simulink model "VC_v1p1"  (R2022b)
settings: Solver=VariableStepAuto  StartTime=0.0  StopTime=inf  FixedStep=1/100  MaxStep=ts  RelTol=1e-3
InitFcn:
  | init_car
  | init_par
values from neighbouring files (symbols this model uses):
  east0 = EWP(1)    [run_VC_bench.m]
  g = 9.81    [init_car.m]
  north0 = NWP(1)    [run_VC_bench.m]
  NUM_WP = length(NWP)    [run_VC_bench.m]
  psi0 = (pi/180)*HWP(1)    [run_VC_bench.m]
  ts = 1/fs    (= 0.01)    [init_car.m]
  vcg0 = 0    [run_VC_bench.m]
  WPT_MTX = [NWP,EWP,HWP,VWP,KWP,SWP]    [run_VC_bench.m]
undefined symbols (not defined in the file or in its folder): car, EWP, NWP, par, ZWP
libraries: simulink x9, matrix_library x6
(part 3 of 3)

== matlab function VC_v1p1/Vehicle_Controller/Lateral Control/Lateral Controller/Calculate control limits/Calculate Curvature Rate and Steering Limits based on vehicle speed using manufacturer data ==
  data: thetadotmax output; thetamax output; delta_s output; kmax output; kpmax output; vcar input; vdead input; ts input; kappa2theta input
function [thetadotmax, thetamax, delta_s, kmax, kpmax] = ...
    speed_based_limits(vcar, vdead, ts, kappa2theta)
%
%  theta = steering wheel angle (deg)
%  delta = front wheel angle (rad)
%  kappa = curvature of path (rad/m)
%
%  thetadotmax = maximumm allowable steering wheel rate (deg/s)
%  thetamax = maximum allowable steering wheel angle (deg)
%  delta_s = distance along path that car moves in one time step (m)
%  kmax = maximum curvature based on published limits (rad/m)
%  kpmax = maximum curvature rate based on published limits (rad/m/m)
%
%  vcar = car velocity (m/s)
%  vdead = deadzone velocity (m/s)
%  ts = sample period (sec)
%  kappa2theta = assumed linear scale factor between kappa and theta

%  This function computes the maximum curvature rate and the max theta at a
%  given vehicle speed based on GM published limits.
%
%  k' = dk/ds [rad/m^2]      vcar = ds/dt [m/s]
%
%  delta[deg] = theta2delta * theta[deg]
%
%  theta[deg] = k2theta * k[rad/m]
%
%  delta[rad] = k2delta * k[rad/m]
%
%  dk    d( theta )      1      (dtheta/dt)        1        (dtheta)
%  -- = ----------- = ------- * ----------- = ----------- * --------
%  ds   ds(k2theta)   k2theta   (  ds/dt  )   k2theta * v   (  dt  )
%
%  Check units:
%     dtheta/dt[deg/sec]
%     k2theta[deg-m/rad] * v[m/s] -> [deg-m^2/rad-s]
%
%  Last Updated:  1/26/2023

%  --initialize local persistent variables

persistent KPH THETAMAX THETADOTMAX NLUT mps2kph

if isempty(KPH)
    %  --define the GM limits on steering rate (lookup tables)
    KPH = [0 15 20 30 35 45 50 65 200];     % kilometers/hour
    THETAMAX = [531 531 475 375 325 235 100 75 10];     % degrees
    THETADOTMAX = [600 600 600 600 400 200 140 95 50];  % degrees/sec
    NLUT = 9;  % number of elements in the LUTs
    
    %  --define the conversion constants
    mps2kph = 3.6;          % kph(ki/hour) = mps2kph * mps(m/s)    
end


%  --evaluate the limits for the input speed

kph = mps2kph * abs(vcar);


%  --interpolate the LUT for the given input speed

if (kph <= KPH(1))
    %  --saturate at the minimum speed in the LUT
    thetadotmax = THETADOTMAX(1);   % (deg/s)
    thetamax = THETAMAX(1);         % (deg)
    
elseif (kph >= KPH(NLUT))
    %  --saturate at the maximum speed in the LUT
    thetadotmax = THETADOTMAX(NLUT);   % (deg/s)
    thetamax = THETAMAX(NLUT);         % (deg)
    
else
    %  --find the interval containing this speed
    index = 2;
    while (kph > KPH(index))
        index = index + 1;  % always points to the upper end of the interval
    end
    
    %  --interpolate the values
    ratio = (kph - KPH(index-1)) / (KPH(index) - KPH(index-1));
    
    thetadotmax = THETADOTMAX(index-1) + ...
        ratio * (THETADOTMAX(index) - THETADOTMAX(index-1));  % (deg/s)
    
    thetamax = THETAMAX(index-1) + ...
        ratio * (THETAMAX(index) - THETAMAX(index-1));  % (deg)
end


%  --compute the maximum curvature based on speed

kmax = thetamax / kappa2theta;


%  --convert thetadotmax (deg/s) to kpmax (rad/m^2)

if (abs(vcar) > 0.1)
    kpmax = thetadotmax / (kappa2theta * vcar);   % (rad/m^2)
else
    %  --saturate to avoid the zero-divide
    kpmax = THETADOTMAX(1) / (kappa2theta * 0.1);   % (rad/m^2);
end


%  --determine how far vehicle traveled in one time step

if (abs(vcar) < vdead)
    %  --car is effectively stopped
    delta_s = 0;
else
    %  --car is moving
    delta_s = abs(vcar) * ts;
end

return

== matlab function VC_v1p1/Vehicle_Controller/Lateral Control/Lateral Controller/Calculate control limits/Calculate Curvature Rate Limits based on geometry ==
  data: kcar input; R input; kpmax_geo output; kpmin_geo output
function [kpmax_geo,kpmin_geo] = geometry_based_limits(kcar, R)
%
%  This is a gateway function to get_kp_limit.m

[kpmax_geo,kpmin_geo] = get_kp_limit(kcar,R);

return

== matlab function VC_v1p1/Vehicle_Controller/Lateral Control/Lateral Controller/Calculate the next desired Curvature Rate ==
  data: kcar input size=1; kpmax input size=1; kpmin input size=1; R input size=1; psi input size=1; Ncar input size=1; Ntarget input size=1; Ecar input size=1; Etarget input size=1; kpdes output size=1
function kpdes = optimal_curvature_rate(kcar, kpmax, kpmin, R, ...
    psi, Ncar, Ntarget, Ecar, Etarget)

%  This is a gateway function to get_opt_curvature_rate.m

maxiter = 10;
tol = 1e-3;

kpdes  = get_opt_curvature_rate(kcar, kpmax, kpmin, R, ...
    psi, Ncar, Ntarget, Ecar, Etarget, maxiter, tol);

return

== matlab function VC_v1p1/Vehicle_Controller/Longitudinal Control/Longitudinal Controller/velocity feedback pre-processor/MATLAB Function ==
  data: speed_mode input; vref input; vcar input; vdes output; alat input; along input; ts input; max_speed input; max_alat input; fbreak_vref input; verror output; vdead input; car_is_stopped output
function [vdes,verror,car_is_stopped]  = prefilter_vref(speed_mode, ...
    vref,vcar,alat,along, ...
    ts,max_speed,max_alat,fbreak_vref,vdead)

%  vdes = final desired reference velocity for control (m/s)
%  verror = velocity error for control (m/s)
%  car_is_stopped = boolean indicating that the car is not moving
%
%  speed_mode = operating mode for speed control
%    * = both torque and brake commands are set to zero
%    1 = brake hold mode (max brake and no torque)
%    2 = use internal torque and brake signals
%    3 = use external torque and brake signals
%  vcar = current car velocity (m/s)
%  vref = current input reference velocity (m/s)
%  alat = current lateral acceleration (m/s/s)
%  along = current longitudinal acceleration (m/s/s) [not yet used]
%  ts = sample period (sec)
%  max_speed = maximum vehicle speed (m/s)
%  max_alat = maximum lateral acceleration (m/s/s)
%  fbreak_vref = break frequency (Hz) of 1st order low-pass filter
%  vdead = deadzone velocity (m/s)

%  --define persistent local variables
persistent VDES VERROR LAST_SPEED_MODE LPFA LPFB CAR_IS_STOPPED
persistent VREF LAST_VREF_IN LAST_VREF_OUT
persistent LAST_ALAT_IN LAST_ALAT_OUT
persistent soft_start_state deltaVREF startup_accel soft_start_count
if (isempty(VDES))
    VDES = 0;
    VERROR = 0;
    CAR_IS_STOPPED = 1;
    LAST_SPEED_MODE = 0;
    VREF = 0;
    LAST_VREF_IN = 0;
    LAST_VREF_OUT = 0;
    LAST_ALAT_IN = 0;
    LAST_ALAT_OUT = 0;
    soft_start_state = 0;
    startup_accel = 0.5;  % m/s/s
    deltaVREF = startup_accel * ts;
    soft_start_count = 0;

    %  --compute low-pass vref filter coefficients
    w = 2*pi*fbreak_vref;   % break frequency for vref (rad/s)
    LPFA = (w*ts-2)/(w*ts+2);  % numerator coefficient
    LPFB = (w*ts)/(w*ts+2);    % denominator coefficient
end

%  --check for a mode transition
if (speed_mode ~= LAST_SPEED_MODE)
    %  --recompute low-pass vref filter coefficients
    w = 2*pi*fbreak_vref;   % break frequency for vref (rad/s)
    LPFA = (w*ts-2)/(w*ts+2);  % numerator coefficient
    LPFB = (w*ts)/(w*ts+2);    % denominator coefficient

    %  --reset local signals
    VDES = 0;
    VERROR = 0;
    CAR_IS_STOPPED = 1;
    VREF = 0;
    LAST_VREF_IN = 0;
    LAST_VREF_OUT = 0;
    LAST_ALAT_IN = 0;
    LAST_ALAT_OUT = 0;
    soft_start_state = 0;
    deltaVREF = startup_accel * ts;
    soft_start_count = 0;
end


%  --check to see if car is moving
if (abs(vcar) < vdead)
    %  --car is not moving
    CAR_IS_STOPPED = 1;
else
    %  --car is still moving
    CAR_IS_STOPPED = 0;
end


%  --only process for mode 2 (autonomous speed control)
if (speed_mode == 2)
    %  --filter the absolute lateral acceleration input
    alat_out = LPFB * (abs(alat) + LAST_ALAT_IN) - LPFA * LAST_ALAT_OUT;
    LAST_ALAT_OUT = alat_out;
    LAST_ALAT_IN = abs(alat);


    %  --adjust the upper speed limit based on lateral acceleration
    if (CAR_IS_STOPPED == 1)
        %  --car is not moving so just use max speed
        vmax = max_speed;
        soft_start_count = 0;  % reset soft_start counter

    else
        %  --car is moving so check lateral acceleration limit
        if (abs(alat_out) > max_alat)
            %  --lat acceleration exceeded limits (too high)
            %    calculate vmax based on max alat
            %    (vmax/vcar)^2 = (max_alat/alat)
            vmax = abs(vcar) * sqrt(max_alat / abs(alat_out));

            if (vmax > max_speed)
                %  --saturate the velocity limit at the max speed limit
                vmax = max_speed;
            end
        else
            %  --lat acceleration is within limits
            vmax = max_speed;
        end
    end


    %  --soft start state machine
    switch soft_start_state
        case 0  %  --waiting for start
            if (vref > 0)
                %  --enter soft-start mode
                VREF = 0;
                soft_start_state = 2;
            end

            LAST_VREF_IN = VREF;
            LAST_VREF_OUT = VREF;
            soft_start_count = 0;

        case 1  %  --ramp up the ref velocity at a fixed rate for 1 sec
            if (soft_start_count < 200)
                %  --counter has not yet expired
                VREF = VREF + deltaVREF;
                soft_start_count = soft_start_count + 1;
            else
                %  --counter has expired
                soft_start_state = 2;
            end

        case 2  %  --ramp up the reference velocity at a fixed rate
            if (VREF < min(vref,vmax))
                %  --reference velocity is still below the command
                VREF = VREF + deltaVREF;
            else
                %  --reference velocity has reached the command
                soft_start_state = 3;
            end

        case 3  %  --track the actual reference input velocity now
            if (CAR_IS_STOPPED == 1)
                %  --return to wait state
                soft_start_state = 0;
            else
                %  --normal operation
                VREF = min(vref,vmax);
            end

        otherwise
            %  --should not be here
            soft_start_state = 0;
    end


    %  --low-pass filter the reference velocity
    VDES = LPFB * (VREF + LAST_VREF_IN) - LPFA * LAST_VREF_OUT;
    LAST_VREF_OUT = VDES;  % desired reference velocity
    LAST_VREF_IN = VREF;


    %  --compute the velocity feedback error for control
    VERROR = VDES - vcar;

else
    %  --not doing speed control so zero the outputs
    VDES = 0;
    VERROR = 0;
    soft_start_state = 0;
end


%  --transfer outputs
vdes = VDES;
verror = VERROR;
car_is_stopped = CAR_IS_STOPPED;
LAST_SPEED_MODE = speed_mode;

return

== matlab function VC_v1p1/Vehicle_Controller/Lateral Control/Lateral Controller/Calculate Steering Command/Integrate Curvature Rate and compute next Steering Command ==
  data: steer_cmd output; steer_mode input; thetadotmax input; thetamax input; delta_s input; kmax input; kpdes input; kappa2theta input; ts input; max_steer input; min_steer input; max_delta_steer input; kdes output
function [steer_cmd,kdes] = integrate_curv_rate(steer_mode, ...
    thetadotmax, thetamax, delta_s, kmax, kpdes, ...
    kappa2theta, ts, max_steer, min_steer, max_delta_steer)

%  steer_cmd = output steering wheel command position (deg)
%
%  steer_mode = operating mode selector for steering
%    * = steer command set to zero
%    1 = hold steer signal at last value
%    2 = use internal steer signal
%    3 = use external steer signal
%  thetadotmax = maximum steering wheel rate (deg/s)
%  thetamax = maximum steering wheel position (deg)
%  delta_s = distance car travels over one time step (m)
%  kmax = maximum curvature (rad/m)
%  kpdes = desired curvature rate (rad/m/m)
%  kappa2theta = conversion factor between curvature and steering wheel angle
%  ts = sample period (sec)
%  max_steer = maximum allowable steering wheel angle (deg)
%  min_steer = minimum allowable steering wheel angle (deg)
%  max_delta_steer = maximum change in steering wheel command angle (deg)

%  --define local persistent variables
persistent KDES STEER_CMD LAST_STEER_MODE LAST_STEER_CMD
if (isempty(KDES))
    %  --initialize local persistent variables at compile time
    KDES = 0;
    STEER_CMD = 0;
    LAST_STEER_MODE = 0;
    LAST_STEER_CMD = 0;
end


%  --check for steer mode

switch steer_mode
    case 1
        %  --halt the integration, hold output value constant
        % do nothing here

    case 2
        %  --reset integrator on mode transition
        if (steer_mode ~= LAST_STEER_MODE)
            KDES = 0;
        end

        %  --integrate the curvature rate to get the desired curvature
        KDES = KDES + kpdes * delta_s;  % (rad/m)


        %  --saturate the desired curvature
        if (KDES > kmax)
            %  --saturate at upper limit
            KDES = kmax;
        elseif (KDES < -kmax)
            %  --saturate at lower limit
            KDES = -kmax;
        end

    otherwise
        KDES = 0;
end


%  --compute the next steering command
STEER_CMD = KDES * kappa2theta;  % (deg)


%  --compute the max delta steer
MAX_delta_steer = thetadotmax * ts;  % (deg) = (deg/s) * (s)
MAX_delta_steer = min(MAX_delta_steer, max_delta_steer);


%  --rate limit the steering command
if (STEER_CMD > (LAST_STEER_CMD + MAX_delta_steer))
    %  --delta steer is too large in the positive direction
    STEER_CMD = LAST_STEER_CMD + MAX_delta_steer;

elseif (STEER_CMD < (LAST_STEER_CMD - MAX_delta_steer))
    %  --delta steer is too large in the negative direction
    STEER_CMD = LAST_STEER_CMD - MAX_delta_steer;
end


%  --choose conservztive steering command limits
if (thetamax < max_steer)
    MAX_steer = thetamax;
else
    MAX_steer = max_steer;
end
if (min_steer < -thetamax)
    MIN_steer = -thetamax;
else
    MIN_steer = min_steer;
end

%  --saturate the steering command
if (STEER_CMD > MAX_steer)
    STEER_CMD = MAX_steer;
elseif (STEER_CMD < MIN_steer)
    STEER_CMD = MIN_steer;
end


%  --transfer local variables
steer_cmd = STEER_CMD;
kdes = KDES;
LAST_STEER_CMD = steer_cmd;
LAST_STEER_MODE = steer_mode;

return

== matlab function VC_v1p1/Vehicle_Controller/Longitudinal Control/Longitudinal Controller/Speed Controller/PID Controller for tracking speed ==
  data: speed_mode input; torque_cmd output; pitch input; verror input; ts input; max_drv_torque input; max_delta_torque input; min_brk_torque input; max_delta_brake input; kp input; ki input; kd input; kff input; fbreak_diff input; fbreak_fflpf input
function torque_cmd  = speed_controller( ...
    speed_mode,pitch,verror,ts, ...
    max_drv_torque,max_delta_torque, ...
    min_brk_torque,max_delta_brake, ...
    kp,ki,kd,kff,fbreak_diff,fbreak_fflpf)

%  torque_cmd = final output torque command (Nm)
%
%  speed_mode = operating mode for speed control
%    * = both torque and brake commands are set to zero
%    1 = brake hold mode (max brake and no torque)
%    2 = use internal torque and brake signals
%  pitch = pitch angle of the vehicle (rad)
%  verror = velocity error for speed control (m/s)
%  ts = sample period (sec)
%  max_drv_torque = maximum allowable drive torque (Nm)
%  min_drv_torque = minimum allowable drive torque (Nm)
%  max_delta_torque = maximum allowable change in drive torque (Nm)
%  max_brk_torque = maximum allowable brake torque (Nm)
%  min_brk_torque = minimum allowable brake torque (Nm)
%  max_delta_brake = maximum allowable change in brake torque (Nm)
%  kp = proportional feedback gain
%  ki = integral feedback gain
%  kd = derivative feedback gain
%  kff = feedforward gain for pitch angle compensation
%  fbreak_diff = 1st order break frequency (Hz) for differentiator
%  fbreak_fflpf = 1st order break frequency (Hz) for feedforward LPF

%  --define the local persistent variables
persistent LPFA LPFB DIFFA DIFFB PROP_ERROR INTE_ERROR DERIV_ERROR
persistent LAST_SPEED_MODE LAST_TORQUE_CMD
persistent LAST_VERROR LAST_PITCH PITCH_OUT
if (isempty(LAST_SPEED_MODE))
    %  --initialize local persistent variables
    LAST_SPEED_MODE = 0;
    PROP_ERROR = 0;
    INTE_ERROR = 0;
    DERIV_ERROR = 0;
    LAST_VERROR = 0;
    LAST_PITCH = 0;
    PITCH_OUT = 0;
    LAST_TORQUE_CMD = 0;

    %  --compute low-pass (pitch) filter coefficients
    w = 2*pi*fbreak_fflpf;       % break frequency for vref (rad/s)
    LPFA = (w*ts-2)/(w*ts+2);  % numerator coefficient
    LPFB = (w*ts)/(w*ts+2);    % denominator coefficient

    %  --compute the high-pass (differentiator) filter coefficients
    w = 2*pi*fbreak_diff;       % break frequency (rad/s)
    DIFFA = (w*ts-2)/(w*ts+2);  % discrete-time denominator coefficient
    DIFFB = (2*w)/(w*ts+2);     % discrete-time numerator coefficient
end


%  --check for a mode transition
if (speed_mode ~= LAST_SPEED_MODE)
    %  --recompute low-pass (pitch) filter coefficients
    w = 2*pi*fbreak_fflpf;       % break frequency for vref (rad/s)
    LPFA = (w*ts-2)/(w*ts+2);  % numerator coefficient
    LPFB = (w*ts)/(w*ts+2);    % denominator coefficient

    %  --recompute the high-pass (differentiator) filter coefficients
    w = 2*pi*fbreak_diff;       % break frequency (rad/s)
    DIFFA = (w*ts-2)/(w*ts+2);  % discrete-time denominator coefficient
    DIFFB = (2*w)/(w*ts+2);     % discrete-time numerator coefficient

    %  --reset local persistent variables
    PROP_ERROR = 0;
    INTE_ERROR = 0;
    DERIV_ERROR = 0;
    LAST_VERROR = 0;
    LAST_PITCH = 0;
    PITCH_OUT = 0;
    LAST_TORQUE_CMD = 0;
end


%  --only process for mode 2 (autonomous speed control)
if (speed_mode == 2)
    %  --evaluate the proportional control term
    PROP_ERROR = kp * verror;


    %  --evaluate and saturate the integral control term
    INTE_ERROR = INTE_ERROR + ki * verror;
    if (INTE_ERROR > max_drv_torque)
        %  --extreme upper limit
        INTE_ERROR = max_drv_torque;
    elseif (INTE_ERROR < min_brk_torque)
        %  --extreme lower limit
        INTE_ERROR = min_brk_torque;
    end


    %  --evaluate the derivative control term
    DERIV_ERROR = (kd * DIFFB * (verror - LAST_VERROR)) - DIFFA * DERIV_ERROR;
    LAST_VERROR = verror;


    %  --low-pass filter the pitch angle
    PITCH_OUT = LPFB * (pitch - LAST_PITCH) - LPFA * PITCH_OUT;
    LAST_PITCH = pitch;

    
    %  --compute the total PID control signal with FF pitch compensation
    TORQUE_CMD = PROP_ERROR + INTE_ERROR + DERIV_ERROR + kff * sin(PITCH_OUT);


    %  --rate limit the TORQUE_CMD value
    if (TORQUE_CMD > 0)
        %  --use throttle torque limits
        if (TORQUE_CMD > (LAST_TORQUE_CMD + max_delta_torque))
            %  --delta torque is too large in the positive direction
            TORQUE_CMD = LAST_TORQUE_CMD + max_delta_torque;

%         elseif (TORQUE_CMD < (LAST_TORQUE_CMD - max_delta_torque))
%             %  --delta torque is too large in the negative direction
%             TORQUE_CMD = LAST_TORQUE_CMD - max_delta_torque;
        end

        %  --saturate the final torque command
        if (TORQUE_CMD > max_drv_torque)
            %  --requested torque exceeds upper limit
            TORQUE_CMD = max_drv_torque;
        end

    else
        %  --use brake torque limits
        if (TORQUE_CMD > (LAST_TORQUE_CMD + max_delta_brake))
            %  --delta torque is too large in the positive direction
            TORQUE_CMD = LAST_TORQUE_CMD + max_delta_brake;

%         elseif (TORQUE_CMD < (LAST_TORQUE_CMD - max_delta_brake))
%             %  --delta torque is too large in the negative direction
%             TORQUE_CMD = LAST_TORQUE_CMD - max_delta_brake;
        end
        
        %  --saturate the final torque command
        if (TORQUE_CMD < min_brk_torque)
            %  --requested torque exceeds upper limit
            TORQUE_CMD = min_brk_torque;
        end

    end

else
    %  --all other speed_mode values have zero torque output
    TORQUE_CMD = 0;
end


%  --save the previous local TORQUE_CMD and BRAKE_CMD values
LAST_TORQUE_CMD = TORQUE_CMD;
LAST_SPEED_MODE = speed_mode;


%  --transfer local signals to the outputs
torque_cmd = TORQUE_CMD;

return

== matlab function VC_v1p1/Vehicle_Controller/Longitudinal Control/Longitudinal Controller/Speed Controller/Compensate brake path ==
  data: speed_mode input; torque_cmd input; throttle_cmd output; ts input; wT input; zT input; wB input; zB input; brake_cmd output; min_brk_torque input
function [throttle_cmd,brake_cmd] = lead_compensator(speed_mode, ...
    torque_cmd, ts, wT, zT, wB, zB, min_brk_torque)

%  throttle_cmd = final torque (throttle) command signal (Nm)
%  brake_cmd = lead-compensated brake command signal (Nm)
%
%  speed_mode = operating mode for speed control
%  torque_cmd = net input throttle command (Nm)
%  ts = sample period (sec)
%  wT = 2nd order natural frequency (rad/s) of torque dynamics
%  zT = damping ratio of torque dynamics
%  wB = 2nd order natural frequency (rad/s) of brake dynamics
%  zB = damping ratio of brake dynamics


%  --define  local persistent variables
persistent LAST_SPEED_MODE B0 B1 B2 A1 A2 ykm1 ykm2 ukm1 ukm2
persistent THROTTLE_CMD BRAKE_CMD
if (isempty(LAST_SPEED_MODE))
    %  --initialize local persistent variables
    LAST_SPEED_MODE = 0;
    ykm1 = 0;
    ykm2 = 0;
    ukm1 = 0;
    ukm2 = 0;
    THROTTLE_CMD = 0;
    BRAKE_CMD = 0;

    %  --initialize lead filter coefficients
    A0 = wB^2*(4*ts*wT*zT + ts^2*wT^2 + 4);
    A1 = wB^2*(2*ts^2*wT^2 - 8) / A0;
    A2 = wB^2*(ts^2*wT^2 - 4*ts*wT*zT + 4) / A0;
    B0 = wT^2*(4*ts*wB*zB + ts^2*wB^2 + 4) / A0;
    B1 = wT^2*(2*ts^2*wB^2 - 8) / A0;
    B2 = wT^2*(ts^2*wB^2 - 4*ts*wB*zB + 4) / A0;
end


%  --check for a mode change
if (speed_mode ~= LAST_SPEED_MODE)
    %  --reinitialize local persistent variables
    ykm1 = 0;
    ykm2 = 0;
    ukm1 = 0;
    ukm2 = 0;
    THROTTLE_CMD = 0;
    BRAKE_CMD = 0;

    %  --initialize lead filter coefficients
    A0 = wB^2*(4*ts*wT*zT + ts^2*wT^2 + 4);
    A1 = wB^2*(2*ts^2*wT^2 - 8) / A0;
    A2 = wB^2*(ts^2*wT^2 - 4*ts*wT*zT + 4) / A0;
    B0 = wT^2*(4*ts*wB*zB + ts^2*wB^2 + 4) / A0;
    B1 = wT^2*(2*ts^2*wB^2 - 8) / A0;
    B2 = wT^2*(ts^2*wB^2 - 4*ts*wB*zB + 4) / A0;
end


%  --only process torque/brake split when mode=2 (autonomous speed)

if (speed_mode == 1)
    %  --apply max brake torque in RDY_BRAKE mode
    BRAKE_CMD = min_brk_torque;
    THROTTLE_CMD = 0;

elseif (speed_mode == 2)
    %  --determine if torque input is for throttle or brake
    if (torque_cmd > 0)
        %  --process input torque_cmd as a throttle command
        THROTTLE_CMD = torque_cmd;
        BRAKE_CMD = 0;
        ykm1 = 0;
        ykm2 = 0;
        ukm1 = 0;
        ukm2 = 0;

    else
        %  --process input torque_cmd as a brake command
        THROTTLE_CMD = 0;

        %  --evaluate the lead filter with the next brake_cmd input
        BRAKE_CMD = - A1*ykm1 - A2*ykm2 + B0*torque_cmd + B1*ukm1 + B2*ukm2;

        %  --saturate the lead filter output (brake_cmd can never be positive)
        if (BRAKE_CMD > 0), BRAKE_CMD = 0; end

        %  --shift data for the next time step
        ykm2 = ykm1;
        ykm1 = BRAKE_CMD;   % previous output
        ukm2 = ukm1;
        ukm1 = torque_cmd;  % previous input
    end

else
    %  --zero all internal states and outputs
    ykm1 = 0;
    ykm2 = 0;
    ukm1 = 0;
    ukm2 = 0;
    THROTTLE_CMD = 0;
    BRAKE_CMD = 0;
end


%  --transfer outputs
LAST_SPEED_MODE = speed_mode;
throttle_cmd = THROTTLE_CMD;
brake_cmd = BRAKE_CMD;

return;

== matlab function VC_v1p1/Vehicle_Controller/Lateral Control/Lateral Controller/Calculate Steering Command/MATLAB Function ==
  data: steer_mode input; steer_cmd input; ts input; steer_lead output; fz_lead input; zz_lead input; fp_lead input
function steer_lead = lead_compensator(steer_mode,steer_cmd,ts,...
    fz_lead,zz_lead,fp_lead)
%  This function implements a 3rd order IIR filter using a Direct-Form II
%  structure.  This is a lead filter designed specifically to
%  compensate the steering command signal.
%
%  The Laplace-domain transfer function is:
%
%  y(s)     wp^3     (s^2 + 2*zz*wz*s + wz^2)   -> two complex zeros
%  ---- = -------- * ------------------------
%  x(s)   (s+wp)^3            wz^2              -> three real poles
%
%  The equivalent Z-domain transfer function is:
%
%  y(z)   b0*z^3 + b1*z^2 + b2*z + b3
%  ---- = ---------------------------
%  x(z)     z^3 + a1*z^2 + a2*z + a3
%
%  steer_cmd = input sample to the filter at time step k
%  ts = sample period (sec)
%  fz_lead = 2nd order zero frequency (Hz)
%  zz_lead = 2nd order zero damping ratio (nondim)
%  fp_lead = 1st order pole frequency (Hz)
%  steer_mode = operational mode for steer control
%  steer_lead = output sample from the filter at time step k
%  
%  Last Updated:  1/26/2023

%  --define local persistent variables
persistent LAST_STEER_MODE A1 A2 A3 B0 B1 B2 B3 LAST_STEER_LEAD
persistent ykm1 ykm2 ykm3 ukm1 ukm2 ukm3
if (isempty(LAST_STEER_MODE))
    %  --initialize local persistent variables
    LAST_STEER_MODE = 0;
    LAST_STEER_LEAD = 0;
    ykm1 = 0; ykm2 = 0; ykm3 = 0;
    ukm1 = 0; ukm2 = 0; ukm3 = 0;

    %  --initialize lead filter coefficients
    wz = 2*pi*fz_lead;
    zz = zz_lead;
    wp = 2*pi*fp_lead;

    A0 = (wz^2*(ts*wp + 2)^3);
    A1 = (3*wz^2*(ts*wp - 2)*(ts*wp + 2)^2) / A0;
    A2 = (3*wz^2*(ts*wp - 2)^2*(ts*wp + 2)) / A0;
    A3 = (wz^2*(ts*wp - 2)^3) / A0;
    B0 = (ts*wp^3*(4*ts*wz*zz + ts^2*wz^2 + 4)) / A0;
    B1 = (ts*wp^3*(3*ts^2*wz^2 + 4*ts*wz*zz - 4)) / A0;
    B2 = (-ts*wp^3*(4*ts*wz*zz - 3*ts^2*wz^2 + 4)) / A0;
    B3 = (ts*wp^3*(ts^2*wz^2 - 4*ts*wz*zz + 4)) / A0;
end


%  --check for a mode change
if (steer_mode ~= LAST_STEER_MODE)
    %  --reinitialize local persistent variables
    LAST_STEER_LEAD = 0;
    ykm1 = 0; ykm2 = 0; ykm3 = 0;
    ukm1 = 0; ukm2 = 0; ukm3 = 0;

    %  --initialize lead filter coefficients
    wz = 2*pi*fz_lead;
    zz = zz_lead;
    wp = 2*pi*fp_lead;

    A0 = (wz^2*(ts*wp + 2)^3);
    A1 = (3*wz^2*(ts*wp - 2)*(ts*wp + 2)^2) / A0;
    A2 = (3*wz^2*(ts*wp - 2)^2*(ts*wp + 2)) / A0;
    A3 = (wz^2*(ts*wp - 2)^3) / A0;
    B0 = (ts*wp^3*(4*ts*wz*zz + ts^2*wz^2 + 4)) / A0;
    B1 = (ts*wp^3*(3*ts^2*wz^2 + 4*ts*wz*zz - 4)) / A0;
    B2 = (-ts*wp^3*(4*ts*wz*zz - 3*ts^2*wz^2 + 4)) / A0;
    B3 = (ts*wp^3*(ts^2*wz^2 - 4*ts*wz*zz + 4)) / A0;
end


%  --only implement lead filter when mode=2 (autonomous speed)

if (steer_mode == 2)
    %  --evaluate the lead filter with the next steer_cmd input
    yk = - A1*ykm1 - A2*ykm2  - A3*ykm3 + ...
           B0*steer_cmd + B1*ukm1 + B2*ukm2 + B3*ukm3;

    %  --shift data for the next time step
    ykm3 = ykm2;
    ykm2 = ykm1;
    ykm1 = yk;
    ukm3 = ukm2;
    ukm2 = ukm1;
    ukm1 = steer_cmd;

elseif (steer_mode == 1)
    %  --hold the steering command constant
    yk = LAST_STEER_LEAD;

else
    %  --zero all internal states and outputs
    yk = 0;
    ykm1 = 0; ykm2 = 0; ykm3 = 0;
    ukm1 = 0; ukm2 = 0; ukm3 = 0;
end


%  --transfer outputs
LAST_STEER_MODE = steer_mode;
steer_lead = yk;
LAST_STEER_LEAD = steer_lead;

return;

== matlab function VC_v1p1/Vehicle_Controller/Waypoint Path Analyzer/Waypoint Path Analysis/Estimate closest point on path to vehicle/Estimate key parameters at closest path point ==
  data: path_mode input; northr input; eastr input; wpt_status_change input; wpt_index output; NUM_WP input; NWP input; EWP input; north output; east output; vref output; signal output; VWP input; SWP input; xterr output
function [wpt_index,north,east,vref,signal,xterr] = ...
    get_info_at_closest_point(path_mode,northr,eastr, ...
    wpt_status_change,NUM_WP,NWP,EWP,VWP,SWP)

%  This function determines the point on a collection of line segments
%  defined by waypoint vectors NWP and EWP that is closest to the input
%  coordinate (northr,eastr), and determines all local info for that point.
%  
%  path_mode = mode selection for enabling/disabling path computations
%       0 = disable path analysis
%       1 = enable path analysis
%  northr = north-dir coordinate of current vehicle position
%  eastr = east-dir coordinate of current vehicle position
%  wpt_status_change = Boolean indicating that waypoints have changed
%  NUM_WP = total number of valid waypoints in buffers
%  NWP = north-dir coordinate vector of waypoints
%  EWP = east-dir coordinate vector of waypoints
%  VWP = vector of desired velocities at each waypoint
%  SWP = vector of desired bitfield signal at each waypoint
%
%  wpt_index = current index of waypoint closest to (northr,eastr)
%  north = north-dir coordinate of point on segment closest to (northr,eastr)
%  east = east-dir coordinate of point on segment closest to (northr,eastr)
%  vref = reference velocity at closest point
%  signal = bitfield signal at closest point
%  xterr = cross-track error (lateral distance between car and path)
%
%  This function calls the following handcoded functions:
%       nearest_point_to_wpts.m
%
%  Last Modified:  2/18/2023

%  --define local persistent variables
persistent WPT_INDEX NORTH EAST VREF SIGNAL XTERR
if (isempty(WPT_INDEX))
    %  --initialize persistent variables
    WPT_INDEX = 1;
    NORTH = NWP(1);
    EAST = EWP(1);
    VREF = 0;
    SIGNAL = 0;
    XTERR = 0;
end


%  --check to see if waypoint analysis has been enabled
if ((path_mode == 1) && (NUM_WP > 0))
    %  --check to see if the waypoints have been updated
    if (wpt_status_change)
        %  --reset starting index for search
        WPT_INDEX = 1;
    end

    %  --find the closest point on the path
    [WPT_INDEX,NORTH,EAST,uc,XTERR,ds] = ...
        nearest_point_to_wpts(WPT_INDEX,northr,eastr,NUM_WP,NWP,EWP);


    %  --interpolate the desired velocity at the closest point
    if ((uc > ds) && (WPT_INDEX == (NUM_WP-1)))
        %  --beyond the last waypoint, saturate at last value
        VREF = VWP(WPT_INDEX+1);

    elseif ((uc < 0) && (WPT_INDEX == 1))
        %  --prior to the first waypoint, saturate at first value
        VREF = VWP(WPT_INDEX);

    else
        %  --interior point of waypoints
        VREF = VWP(WPT_INDEX) + (VWP(WPT_INDEX+1)-VWP(WPT_INDEX))*(uc/ds);
    end


    %  --extract the signal bitfield for the closest point
    SIGNAL = SWP(WPT_INDEX);
    

else  % --analysis has been disabled
    %  --reset persistent variables
    WPT_INDEX = 1;
    NORTH = NWP(1);
    EAST = EWP(1);
    VREF = 0;
    SIGNAL = 0;
    XTERR = 0;
end


%  --transfer outputs
wpt_index = WPT_INDEX;
north = NORTH;
east = EAST;
vref = VREF;
signal = SIGNAL;
xterr = XTERR;

return

== matlab function VC_v1p1/Vehicle_Controller/Waypoint Path Analyzer/Waypoint Path Analysis/Estimate lookahead target point/MATLAB Function ==
  data: path_mode input; wpt_index input; northc input; eastc input; target_index output; minLA input; maxLA input; NUM_WP input; NWP input; EWP input; northt output; eastt output
function [target_index,northt,eastt] = lookahead_target( ...
    path_mode,wpt_index,northc,eastc,minLA,maxLA,NUM_WP,NWP,EWP)

%  This function determines the point on a collection of line segments
%  defined by waypoint vectors NWP and EWP that is approximately at a
%  specified lookahead target distance.
%
%  path_mode = mode indicating whether path analysis is enabled or disabled
%  wpt_index = index of current waypoint closest to car
%  northc = north-dir coordinate of initial path point
%  eastc = east-dir coordinate of initial path point
%  minLA = minimum lookahead distance from initial point to target
%  maxLA = maximum lookahead distance from initial point to target
%  NUM_WP = number of valid waypoints in vectors
%  NWP = north-dir coordinate vector of waypoints
%  EWP = east-dir coordinate vector of waypoints
%
%  target_index = index of waypoint closest to (northt,eastt)
%  northt = north-dir coordinate of target point on waypoint path
%  eastt = east-dir coordinate of target point on waypoint path
%
%  This function does not call any handcoded functions.
%
%  Last Modified:  2/19/2023

%  --define local persistent variables
persistent TARGET_INDEX NORTHT EASTT
if (isempty(TARGET_INDEX))
    %  --initialize local persistent variables
    TARGET_INDEX = 1;
    NORTHT = 0;
    EASTT = 0;
end


%  --check to see if path analysis is enabled
if ((path_mode == 1) && (NUM_WP > 0))
    %  --path analysis mode is enabled and we have waypoints

    %  --determine the path heading angle where we currently are

    if (wpt_index == NUM_WP)
        stindex = wpt_index - 1;
    else
        stindex = wpt_index;
    end

    deltaN = NWP(stindex+1) - NWP(stindex);
    deltaE = EWP(stindex+1) - EWP(stindex);

    psi = atan2(deltaE,deltaN);  % path heading [radians]
    

    %  --project out to the lookahead point

    lookahead = 5;  % temporary fixed lookahead distance

    north_lookahead = northc + lookahead * cos(psi);
    east_lookahead = eastc + lookahead * sin(psi);


    %  --find the nearest waypoint to this lookahead

    [TARGET_INDEX,NORTHT,EASTT,~,~,~] = ...
        nearest_point_to_wpts(wpt_index,north_lookahead,east_lookahead,NUM_WP,NWP,EWP);
end

%  --transfer the outputs
target_index = TARGET_INDEX;
northt = NORTHT;
eastt = EASTT;

return

== matlab function VC_v1p1/Vehicle_Controller/Pack Data Log Message/Estimate Jerk/Jerk Estimation Filter ==
  data: mode_select input; alat input; along input; ts input; jlat output; jlong output
function [jlat,jlong] = jerk_differentiator(mode_select,alat,along,ts)
%  This function implements a 3rd order IIR differentiator using a 
%  Direct-Form II structure.  This differentiator is designed specifically
%  to estimate jerk from lateral and longitudinal acceleration inputs.
%
%  See jerk_estimation_vt.pdf for detailed derivation.
%
%  The Laplace-domain transfer function is:
%
%  y(s)   w1 * s             w0^2             -> zero at origin
%  ---- = ------ * ------------------------
%  u(s)   (s+w1)   (s^2 + 2*z0*w0*s + w0^2)   -> three poles
%
%  The equivalent Z-domain transfer function is:
%
%  y(z)   b0*(z^3 + z^2 - z - 1)
%  ---- = ------------------------
%  u(z)   z^3 + a1*z^2 + a2*z + a3
%
%  mode_select = mode selection for resetting filter parameters
%  alat = input lateral acceleration at time step k
%  along = input longitudinal acceleration at time step k
%  ts = sample period (sec)
%
%  jlat = estimated jerk in the lateral direction
%  jlong = estimated jerk in the longitudinal direction
%  
%  Last Updated:  2/4/2023

%  --define local persistent variables
persistent LAST_MODE_SELECT A1 A2 A3 B0
persistent ykm1lat ykm2lat ykm3lat ukm1lat ukm2lat ukm3lat
persistent ykm1lon ykm2lon ykm3lon ukm1lon ukm2lon ukm3lon

if (isempty(LAST_MODE_SELECT))
    %  --initialize local persistent variables
    LAST_MODE_SELECT = 0;
    ykm1lat = 0; ykm2lat = 0; ykm3lat = 0;
    ukm1lat = 0; ukm2lat = 0; ukm3lat = 0;

    ykm1lon = 0; ykm2lon = 0; ykm3lon = 0;
    ukm1lon = 0; ukm2lon = 0; ukm3lon = 0;

    %  --initialize lead filter coefficients (DO NOT CHANGE)
    w0 = 2*pi*10;   % 2nd order break frequency (hardcoded)
    z0 = 0.35;      % 2nd order damping ratio (hardcoded)
    w1 = 2*pi*7;    % 1st order break frequency (hardcoded)

    A0 = ((ts*w1 + 2)*(4*ts*w0*z0 + ts^2*w0^2 + 4));
    A1 = ((ts*w1 - 2)*(4*ts*w0*z0 + ts^2*w0^2 + 4) + (2*ts^2*w0^2 - 8)*(ts*w1 + 2)) / A0;
    A2 = ((ts*w1 + 2)*(ts^2*w0^2 - 4*ts*w0*z0 + 4) + (2*ts^2*w0^2 - 8)*(ts*w1 - 2)) / A0;
    A3 = ((ts*w1 - 2)*(ts^2*w0^2 - 4*ts*w0*z0 + 4)) / A0;
    B0 = (2*ts^2*w0^2*w1) / A0;
end


%  --check for a mode change
if (mode_select ~= LAST_MODE_SELECT)
    %  --reinitialize local persistent variables
    ykm1lat = 0; ykm2lat = 0; ykm3lat = 0;
    ukm1lat = 0; ukm2lat = 0; ukm3lat = 0;

    ykm1lon = 0; ykm2lon = 0; ykm3lon = 0;
    ukm1lon = 0; ukm2lon = 0; ukm3lon = 0;

    %  --initialize differentiator filter coefficients (DO NOT CHANGE)
    w0 = 2*pi*10;   % 2nd order break frequency (hardcoded)
    z0 = 0.35;      % 2nd order damping ratio (hardcoded)
    w1 = 2*pi*7;    % 1st order break frequency (hardcoded)

    A0 = ((ts*w1 + 2)*(4*ts*w0*z0 + ts^2*w0^2 + 4));
    A1 = ((ts*w1 - 2)*(4*ts*w0*z0 + ts^2*w0^2 + 4) + (2*ts^2*w0^2 - 8)*(ts*w1 + 2)) / A0;
    A2 = ((ts*w1 + 2)*(ts^2*w0^2 - 4*ts*w0*z0 + 4) + (2*ts^2*w0^2 - 8)*(ts*w1 - 2)) / A0;
    A3 = ((ts*w1 - 2)*(ts^2*w0^2 - 4*ts*w0*z0 + 4)) / A0;
    B0 = (2*ts^2*w0^2*w1) / A0;
end


%  --differentiate the next lateral acceleration input
yk = - A1*ykm1lat - A2*ykm2lat  - A3*ykm3lat + ...
    B0*(alat + ukm1lat - ukm2lat - ukm3lat);

%  --shift data for the next time step
ykm3lat = ykm2lat;
ykm2lat = ykm1lat;
ykm1lat = yk;
ukm3lat = ukm2lat;
ukm2lat = ukm1lat;
ukm1lat = alat;


%  --differentiate the next longitudinal acceleration input
zk = - A1*ykm1lon - A2*ykm2lon  - A3*ykm3lon + ...
    B0*(along + ukm1lon - ukm2lon - ukm3lon);

%  --shift data for the next time step
ykm3lon = ykm2lon;
ykm2lon = ykm1lon;
ykm1lon = zk;
ukm3lon = ukm2lon;
ukm2lon = ukm1lon;
ukm1lon = along;


%  --transfer outputs
LAST_MODE_SELECT = mode_select;
jlat = yk;
jlong = zk;

return;

== matlab function VC_v1p1/CAN Driver/MATLAB Function ==
  data: AV_mode_active output; AV_start_request input; torque_cmd output; mode_select input; torque_in input; brake_in input; steer_in input; signal_in input; brake_cmd output; steer_cmd output; gear_cmd output
function [AV_mode_active,torque_cmd,brake_cmd,steer_cmd,gear_cmd] = send_CAN_cmds( ...
    AV_start_request,mode_select,torque_in,brake_in,steer_in,signal_in)

%  --define local persistent variables
persistent COUNTER MAXDELAY AV_MODE_ACTIVE
if (isempty(COUNTER))
    COUNTER = 1;
    MAXDELAY = 7;  % number of samples to delay startup request (fake)
    AV_MODE_ACTIVE = 0;
end


%  --check for an AV startup request
if ((AV_start_request == 1) && (mode_select > 0))
    %  --we have a valid request to start
    if (AV_MODE_ACTIVE == 0)
        %  --increment the counter
        COUNTER = COUNTER + 1;

        %  --generate a fake delay to emulate startup
        if (COUNTER >= MAXDELAY)
            %  --we have reached the end of the delay
            COUNTER = 0;
            AV_MODE_ACTIVE = 1;
        end
    end
end


%  --transfer outputs
AV_mode_active = AV_MODE_ACTIVE;
torque_cmd = torque_in;
brake_cmd = brake_in;
steer_cmd = steer_in;
gear_cmd = 1;

return

== matlab function VC_v1p1/Road Grade/MATLAB Function ==
  data: wpt_index input; NWP input; EWP input; grade_rad output; ZWP input
function grade_rad = estimate_grade(wpt_index,NWP,EWP,ZWP)

%   --range check the wpt_index value
N = length(ZWP);
if (wpt_index > N)
    k = N - 1;
else
    k = wpt_index;
end


%  --compute the distance between current and next waypoints
dx = NWP(k+1) - NWP(k);
dy = EWP(k+1) - EWP(k);
dz = ZWP(k+1) - ZWP(k);

ds = sqrt(dx^2 + dy^2);


%  --compute the grade (radians)
grade_rad = atan2(dz,ds);

return

== matlab function VC_v1p1/Chevy Bolt EUV 2023 and GNSS/engine-steer-brake and inertial dynamics/Net Force Applied at CG/MATLAB Function ==
  data: Fsum input; Vdead input; vcg input; Fnet output; Fbrake input
function Fnet  = stick_slip_logic(Fsum,Vdead,vcg,Fbrake)

%  Note:  This code assumes the car will NEVER be driven in reverse.  This
%  function needs to change if the simulation is to ever be used with a car
%  that can go in reverse.

%  --check to see if the car is moving or not

if (vcg > Vdead)
    %  --car has positive velocity (i.e. moving forward)
    %  This is the normal case where the car is moving so the net applied
    %  force is just the sum of all forces

    Fnet = Fsum + Fbrake;

else
    %  --car effectively has zero (or negative) velocity
    %  Due to the fact that brake forces cannot put energy into the system
    %  (i.e. they are non-conservative forces), the effective brake force
    %  will be different than the externally commanded brake force, which
    %  causes the net applied force to be different.  This logic simulates
    %  the real-world effect where a car will actually stop moving even if
    %  a large brake force is applied, and the car will not move backward
    %  if a large brake force is applied.

    if (abs(Fsum) > abs(Fbrake))
        %  --we have a net non-zero applied force
        %  This allows the car to start moving again when enough force is
        %  applied while the vehicle is at zero velocity, i.e. the car will
        %  not get "stuck" in this stopped state.

        Fnet = Fsum + Fbrake;

    else
        %  --brake force exceeds Fsum, so just set the net force to zero
        %  which is equivalent to choosing a brake force that is whatever
        %  value (less than the input Fbrake value) that is required to
        %  match Fsum such that (Fsum + Fbrake) = 0

        Fnet = 0;
        
    end
end

== matlab function VC_v1p1/Path Planner Emulator/Waypoint Handshake ==
  data: action_select input; new_wpts output; wpt_index input; NUM_WPT_FULL input; WPT_MTX_FULL input; num_wp output; wpt_mtx output
function [new_wpts,num_wp,wpt_mtx] = wpt_handshake( ...
    action_select,wpt_index,NUM_WPT_FULL,WPT_MTX_FULL)

%  --initialize local persistent variables
persistent NEW_WPTS NUM_WP WPT_MTX STATE KSTART KEND MAX_WPTS
if isempty(STATE)
    STATE = 0;
    NEW_WPTS = 0;
    NUM_WP = 0;  % number of valid waypoints in wpt_mtx
    MAX_WPTS = 1024;
    WPT_MTX = zeros(1024,6);
    KSTART = 1;
    KEND = 1;
end


%  --waypoint handshake state machine
switch STATE
    case 0  %  --wait for init_auto action select
        if (action_select == 1)
            NEW_WPTS = 0;  % keep this deasserted until ready
            KSTART = 1;    % set the starting index
            STATE = 1;     % proceed to the next state
        end

    case 1  %  --prepare the next batch of waypoints
        %  --assume we have a full batch (MAX_WPTS) available
        %    then determine the ending waypoint index
        KEND = KSTART + MAX_WPTS - 1;


        %  --check to see if the assumption was valid
        if (KEND > NUM_WPT_FULL)
            %  --the full wpt_mtx does not have enough points remaining
            KEND = NUM_WPT_FULL;
        end


        %  --populate the next wpt_mtx array
        NUM_WP = KEND - KSTART + 1;
        for n = 1:NUM_WP
            index = KSTART + n - 1; % start at KSTART, end at KEND
            WPT_MTX(n,:) = WPT_MTX_FULL(index,:);
        end

        %  --toggle the new_wpts indicator
        if (NEW_WPTS == 0)
            NEW_WPTS = 1;
        else
            NEW_WPTS = 0;
        end

        %  --proceed to the next state
        STATE = 2;


    case 2  %  --wait for wpt_index to reach the end of this batch
        %  --Note:  wpt_index always starts at 1 for every new batch
        %           KSTART is the starting index in the original matrix
        %           KEND is the ending index in the original matrix
        %
        %           In the example below, the "end" is considered to be
        %           five samples before the actual end of data.  It may
        %           only be necessary to trigger an update based on one
        %           sample before the actual end of data.

        if ((KSTART + wpt_index) >= (KEND-5))
            %  --VC has reached the end of this batch of data

            %  --check to see if there is more data to send
            if (KEND < NUM_WPT_FULL)
                %  --we still have data, so update the new starting index
                KSTART = KEND - 1;

                %  prepare the next batch of data
                STATE = 1;
                
            else
                %  --no data left, so terminate
                STATE = 3;
            end

        end

    case 3  %  --end of data
        %  --Note:  This is a dead-end which can only work for simulation
        %  testing.  A different set of logic is required here to get out
        %  of this state in the real implementation.
end


%  --transfer outputs

new_wpts = NEW_WPTS;
num_wp = NUM_WP;
wpt_mtx = WPT_MTX;

return
